simulink model "Modelo_NL_Ley_de_control_NL_EJE_Q"  (R2017a)
settings: Solver=VariableStepAuto  StartTime=0.0  StopTime=1  MaxStep=1e-4  RelTol=1e-3
values from neighbouring files (symbols this model uses):
  alfa_cu = 3.9e-3    (= 0.0039)    [modelo_global_NL.m]
  beq = bl/r^2 + bm    (= 1.5638971155e-05)    [Evaluacion_polos_5_2_2.m]    (also in modelo_global_NL.m = 1.5e-05)
  Cts = 0.818    [modelo_global_NL.m]
  Jeq = Jl/r^2 + Jm    (= 6.9338269301e-06)    [Evaluacion_polos_5_2_2.m]    (also in modelo_global_NL.m = 5.65588462007e-06)
  LambdaM = 0.01546    [Evaluacion_polos_5_2_2.m]    (also in modelo_global_NL.m)
  Ld = 0.0066    [Evaluacion_polos_5_2_2.m]    (also in modelo_global_NL.m)
  Lq = 0.0058    [Evaluacion_polos_5_2_2.m]    (also in modelo_global_NL.m)
  Pp = 3    [Evaluacion_polos_5_2_2.m]    (also in modelo_global_NL.m)
  Rsref = 1.02    [modelo_global_NL.m]
  Rts_amb = 146.7    [modelo_global_NL.m]
  Tamb = 40    [modelo_global_NL.m]
  Tleq = Tl/r    (= 0.02)    [modelo_global_NL.m]
  Tsref = 40    [modelo_global_NL.m]
  Vqs_nom = 19.596    [modelo_global_NL.m]
undefined symbols (not defined in the file or in its folder): sigbuilder_block
libraries: simulink x2
settings Model: Creator=merem  LastModifiedBy=merem

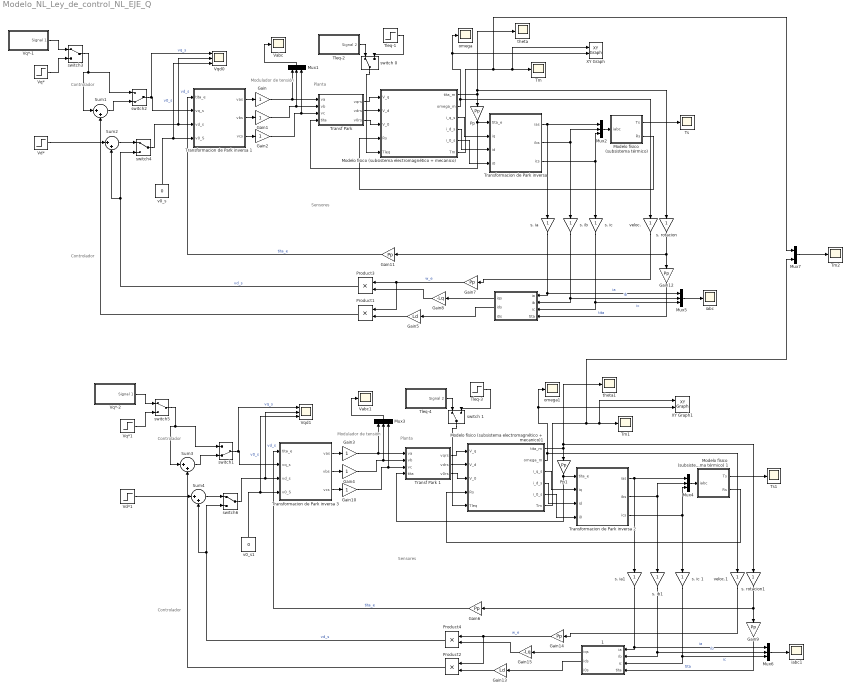
== system Modelo_NL_Ley_de_control_NL_EJE_Q ==
  note: Controlador
  note: Controlador
  note: Modulador de tensión
  note: Sensores
  note: Planta
  note: Controlador
  note: Modulador de tensión
  note: Controlador
  note: Sensores
  note: Planta
  " " : Subsystem
  " 1" : Subsystem
  Gain{,1..4,10} (6 alike) : Gain
  Gain{6..7,9,11..12,14} (6 alike) : Gain  Gain=Pp
  Gain13 : Gain  Gain=Ld
  Gain15 : Gain  Gain=-Lq
  Gain5 : Gain  Gain=Ld
  Gain8 : Gain  Gain=-Lq
  Modelo físico (subsistema electromagnético + mecanico) : Subsystem
  Modelo físico (subsistema electromagnético + mecanico)1 : Subsystem
  "Modelo físico (subsistema térmico) " : Subsystem
  Modelo físico (subsistema térmico) 1 : Subsystem
  Mux{1..6} (6 alike) : Mux  Inputs=3
  Mux7 : Mux  Inputs=2
  Pp : Gain  Gain=Pp
  Pp1 : Gain  Gain=Pp
  Product{1..4} (4 alike) : Product
  Sum{1..4} (4 alike) : Sum  Inputs=|++
  Tleq-1 : Step  Time=0.3  After=Tleq  SampleTime=0
  Tleq-2 : Subsystem  Tag=STV Subsys  LoadFcn=sigbuilder_block('load');  StartFcn=sigbuilder_block('start');  StopFcn=sigbuilder_block('stop');  ClipboardFcn=sigbuilder_block('clipboard');  mask(Sigbuilder block){tuvar=[0:10]}
      mask help: Simulink:masks:SigbuilderBlock_MD
      mask init:
      | if ~strcmp(get_param(bdroot(gcbh),'SimulationStatus'),'stopped') tuvar = sigbuilder_block('maskInit'); end
      settings: CopyFcn=sigbuilder_block('copy');  DeleteFcn=sigbuilder_block('delete');  ModelCloseFcn=sigbuilder_block('modelClose');  PreSaveFcn=sigbuilder_block('preSave');  PauseFcn=sigbuilder_block('pause');  ContinueFcn=sigbuilder_block('continue');  NameChangeFcn=sigbuilder_block('namechange');  OpenFcn=sigbuilder_block('open',[6 30 1012.5 447.75 ]);  CloseFcn=sigbuilder_block('close');
      mask Display: plot(0, 0, 100, 100,[2, 2, 32, 32, 2], [68, 8, 8, 68, 68],[32, 2], [38, 38], [32, 19, 2],[53, 60, 44], [32, 17, 17, 2],[16, 16, 31, 31]);txt = getActiveGroup(gcbh);text(2, 100, txt,'verticalAlignment', 'top');
  Tleq-3 : Step  Time=0.3  After=Tleq  SampleTime=0
  Tleq-4 : Subsystem  Tag=STV Subsys  LoadFcn=sigbuilder_block('load');  StartFcn=sigbuilder_block('start');  StopFcn=sigbuilder_block('stop');  ClipboardFcn=sigbuilder_block('clipboard');  mask(Sigbuilder block){tuvar=[0:10]}
      mask help: Simulink:masks:SigbuilderBlock_MD
      mask init:
      | if ~strcmp(get_param(bdroot(gcbh),'SimulationStatus'),'stopped') tuvar = sigbuilder_block('maskInit'); end
      settings: CopyFcn=sigbuilder_block('copy');  DeleteFcn=sigbuilder_block('delete');  ModelCloseFcn=sigbuilder_block('modelClose');  PreSaveFcn=sigbuilder_block('preSave');  PauseFcn=sigbuilder_block('pause');  ContinueFcn=sigbuilder_block('continue');  NameChangeFcn=sigbuilder_block('namechange');  OpenFcn=sigbuilder_block('open',[6 30 1012.5 447.75 ]);  CloseFcn=sigbuilder_block('close');
      mask Display: plot(0, 0, 100, 100,[2, 2, 32, 32, 2], [68, 8, 8, 68, 68],[32, 2], [38, 38], [32, 19, 2],[53, 60, 44], [32, 17, 17, 2],[16, 16, 31, 31]);txt = getActiveGroup(gcbh);text(2, 100, txt,'verticalAlignment', 'top');
  Tm : Scope
  Tm1 : Scope
  Tm2 : Scope
  "Transf Park " : Subsystem
  Transf Park 1 : Subsystem
  "Transformacion de Park inversa " : Subsystem
  Transformacion de Park inversa 1 : Subsystem
  Transformacion de Park inversa 2 : Subsystem
  Transformacion de Park inversa 3 : Subsystem
  Ts : Scope
  Ts1 : Scope
  Vabc : Scope
  Vabc1 : Scope
  Vd* : Step  Time=0.5  After=1.9596  SampleTime=0
  Vd*1 : Step  Time=0.5  After=1.9596  SampleTime=0
  Vq* : Step  Time=0.1  After=Vqs_nom  SampleTime=0
  Vq*-1 : Subsystem  Tag=STV Subsys  LoadFcn=sigbuilder_block('load');  StartFcn=sigbuilder_block('start');  StopFcn=sigbuilder_block('stop');  ClipboardFcn=sigbuilder_block('clipboard');  mask(Sigbuilder block){tuvar=[0:10]}
      mask help: Simulink:masks:SigbuilderBlock_MD
      mask init:
      | if ~strcmp(get_param(bdroot(gcbh),'SimulationStatus'),'stopped') tuvar = sigbuilder_block('maskInit'); end
      settings: CopyFcn=sigbuilder_block('copy');  DeleteFcn=sigbuilder_block('delete');  ModelCloseFcn=sigbuilder_block('modelClose');  PreSaveFcn=sigbuilder_block('preSave');  PauseFcn=sigbuilder_block('pause');  ContinueFcn=sigbuilder_block('continue');  NameChangeFcn=sigbuilder_block('namechange');  OpenFcn=sigbuilder_block('open',[6 -3.75 1012.5 407.25 ]);  CloseFcn=sigbuilder_block('close');
      mask Display: plot(0, 0, 100, 100,[2, 2, 32, 32, 2], [68, 8, 8, 68, 68],[32, 2], [38, 38], [32, 19, 2],[53, 60, 44], [32, 17, 17, 2],[16, 16, 31, 31]);txt = getActiveGroup(gcbh);text(2, 100, txt,'verticalAlignment', 'top');
  Vq*-2 : Subsystem  Tag=STV Subsys  LoadFcn=sigbuilder_block('load');  StartFcn=sigbuilder_block('start');  StopFcn=sigbuilder_block('stop');  ClipboardFcn=sigbuilder_block('clipboard');  mask(Sigbuilder block){tuvar=[0:10]}
      mask help: Simulink:masks:SigbuilderBlock_MD
      mask init:
      | if ~strcmp(get_param(bdroot(gcbh),'SimulationStatus'),'stopped') tuvar = sigbuilder_block('maskInit'); end
      settings: CopyFcn=sigbuilder_block('copy');  DeleteFcn=sigbuilder_block('delete');  ModelCloseFcn=sigbuilder_block('modelClose');  PreSaveFcn=sigbuilder_block('preSave');  PauseFcn=sigbuilder_block('pause');  ContinueFcn=sigbuilder_block('continue');  NameChangeFcn=sigbuilder_block('namechange');  OpenFcn=sigbuilder_block('open',[6 -3.75 1012.5 407.25 ]);  CloseFcn=sigbuilder_block('close');
      mask Display: plot(0, 0, 100, 100,[2, 2, 32, 32, 2], [68, 8, 8, 68, 68],[32, 2], [38, 38], [32, 19, 2],[53, 60, 44], [32, 17, 17, 2],[16, 16, 31, 31]);txt = getActiveGroup(gcbh);text(2, 100, txt,'verticalAlignment', 'top');
  Vq*1 : Step  Time=0.1  After=Vqs_nom  SampleTime=0
  Vqd0 : Scope  NumInputPorts=3
  Vqd1 : Scope  NumInputPorts=3
  XY Graph : simulink/Sinks/XY Graph  xmin=-0.6  xmax=0.6  ymin=-250  ymax=650  st=-1
  XY Graph1 : simulink/Sinks/XY Graph  xmin=-0.6  xmax=0.6  ymin=-250  ymax=650  st=-1
  iabc : Scope
  iabc1 : Scope
  omega : Scope
  omega1 : Scope
  s. ia : Gain
  s. ia1 : Gain
  s. ib : Gain
  s. ib1 : Gain
  "s. ic " : Gain
  s. ic 1 : Gain
  s. rotacion : Gain
  s. rotacion1 : Gain
  switch 0 : ManualSwitch
  switch 1 : ManualSwitch
  switch1 : ManualSwitch  CurrentSetting=0
  switch2 : ManualSwitch  CurrentSetting=0
  switch{3..6} (4 alike) : ManualSwitch
  theta : Scope
  theta1 : Scope
  v0_s : Constant  Value=0
  v0_s1 : Constant  Value=0
  veloc. : Gain
  veloc.1 : Gain
  wires:
  s. rotacion/1 -> Gain12/1, Gain11/1
  "s. ic "/1 -> Mux5/3, " "/3("ic ")  "ic"
  "Transformacion de Park inversa "/1(ias) -> s. ia/1, Mux2/1
  Gain/1 -> "Transf Park "/1("va "), Mux1/1
  Gain7/1 -> Product1/1, Product3/1  "w_e"
  Gain8/1 -> Product3/2
  Gain1/1 -> "Transf Park "/2(vb), Mux1/2
  s. ia/1 -> Mux5/1, " "/1("ia ")  "ia"
  Gain5/1 -> Product1/2
  Gain2/1 -> "Transf Park "/3(vc), Mux1/3
  Gain12/1 -> " "/4("tita ")  "tita"
  "Transformacion de Park inversa "/3("ics ") -> "s. ic "/1, Mux2/3
  v0_s/1 -> Vqd0/3, Transformacion de Park inversa 1/4("v0_S ")  "v0_s"
  Product3/1 -> Sum2/2, switch4/2  "vd_s"
  s. ib/1 -> Mux5/2, " "/2("ib ")  "ib"
  Gain11/1 -> Transformacion de Park inversa 1/1(tita_e)  "tita_e"
  " "/2("ids ") -> Gain5/1
  Transformacion de Park inversa 1/1(vas) -> Gain/1
  Transformacion de Park inversa 1/3("vcs ") -> Gain2/1
  " "/1(iqs) -> Gain8/1
  "Transformacion de Park inversa "/2(ibs) -> Mux2/2, s. ib/1
  Mux1/1 -> Vabc/1
  Transformacion de Park inversa 1/2(vbs) -> Gain1/1
  Product1/1 -> Sum1/2
  switch2/1 -> Vqd0/1, Transformacion de Park inversa 1/2(vq_s)  "vq_s"
  Sum1/1 -> switch2/2
  "Transf Park "/1(vqrs) -> Modelo físico (subsistema electromagnético + mecanico)/1(V_q)
  "Transf Park "/2("vdrs ") -> Modelo físico (subsistema electromagnético + mecanico)/2(V_d)
  "Transf Park "/3("v0rs ") -> Modelo físico (subsistema electromagnético + mecanico)/3(V_0)
  Pp/1 -> "Transf Park "/4(tita), "Transformacion de Park inversa "/1(tita_e)
  Modelo físico (subsistema electromagnético + mecanico)/1("tita_m ") -> s. rotacion/1, theta/1, Pp/1
  switch3/1 -> Sum1/1, switch2/1
  Vq*/1 -> switch3/2
  Vd*/1 -> Sum2/1
  switch4/1 -> Vqd0/2, Transformacion de Park inversa 1/3(vd_s)  "vd_s"
  Sum2/1 -> switch4/1
  Vq*-1/1(Signal 1) -> switch3/1
  Modelo físico (subsistema electromagnético + mecanico)/3("i_q_s ") -> "Transformacion de Park inversa "/2(iq)
  Modelo físico (subsistema electromagnético + mecanico)/4("i_d_s ") -> "Transformacion de Park inversa "/3(id)
  Modelo físico (subsistema electromagnético + mecanico)/5("i_0_s ") -> "Transformacion de Park inversa "/4(i0)
  Mux2/1 -> "Modelo físico (subsistema térmico) "/1(iabc)
  "Modelo físico (subsistema térmico) "/2(Rs) -> Modelo físico (subsistema electromagnético + mecanico)/4(Rs)
  Tleq-2/1(Signal 2) -> switch 0/1
  Tleq-1/1 -> switch 0/2
  switch 0/1 -> Modelo físico (subsistema electromagnético + mecanico)/5(Tleq)
  "Modelo físico (subsistema térmico) "/1(Ts) -> Ts/1
  Mux5/1 -> iabc/1
  Modelo físico (subsistema electromagnético + mecanico)/2("omega_m ") -> veloc./1, XY Graph/2, omega/1
  veloc./1 -> Gain7/1
  Modelo físico (subsistema electromagnético + mecanico)/6(Tm) -> Mux7/1, XY Graph/1, Tm/1
  Transformacion de Park inversa 2/2(ibs) -> Mux4/2, s. ib1/1
  Transformacion de Park inversa 2/1(ias) -> s. ia1/1, Mux4/1
  Transf Park 1/2("vdrs ") -> Modelo físico (subsistema electromagnético + mecanico)1/2(V_d)
  Transf Park 1/3("v0rs ") -> Modelo físico (subsistema electromagnético + mecanico)1/3(V_0)
  v0_s1/1 -> Vqd1/3, Transformacion de Park inversa 3/4("v0_S ")  "v0_s"
  Sum3/1 -> switch1/2
  Pp1/1 -> Transf Park 1/4(tita), Transformacion de Park inversa 2/1(tita_e)
  Transformacion de Park inversa 3/2(vbs) -> Gain4/1
  Gain14/1 -> Product2/1, Product4/1  "w_e"
  s. ib1/1 -> Mux6/2, " 1"/2("ib ")  "ib"
  Gain13/1 -> Product2/2
  Gain6/1 -> Transformacion de Park inversa 3/1(tita_e)  "tita_e"
  Gain3/1 -> Transf Park 1/1("va "), Mux3/1
  Gain4/1 -> Transf Park 1/2(vb), Mux3/2
  Tleq-3/1 -> switch 1/2
  Sum4/1 -> switch6/1
  Gain9/1 -> " 1"/4("tita ")  "tita"
  Product2/1 -> Sum3/2
  Transformacion de Park inversa 3/1(vas) -> Gain3/1
  Transformacion de Park inversa 3/3("vcs ") -> Gain10/1
  Modelo físico (subsistema electromagnético + mecanico)1/4("i_d_s ") -> Transformacion de Park inversa 2/3(id)
  " 1"/2("ids ") -> Gain13/1
  Mux3/1 -> Vabc1/1
  Tleq-4/1(Signal 2) -> switch 1/1
  switch6/1 -> Vqd1/2, Transformacion de Park inversa 3/3(vd_s)  "vd_s"
  Modelo físico (subsistema electromagnético + mecanico)1/1("tita_m ") -> s. rotacion1/1, theta1/1, Pp1/1
  switch5/1 -> Sum3/1, switch1/1
  Modelo físico (subsistema electromagnético + mecanico)1/3("i_q_s ") -> Transformacion de Park inversa 2/2(iq)
  Vq*-2/1(Signal 1) -> switch5/1
  Transf Park 1/1(vqrs) -> Modelo físico (subsistema electromagnético + mecanico)1/1(V_q)
  Gain15/1 -> Product4/2
  Modelo físico (subsistema térmico) 1/2(Rs) -> Modelo físico (subsistema electromagnético + mecanico)1/4(Rs)
  Product4/1 -> Sum4/2, switch6/2  "vd_s"
  switch 1/1 -> Modelo físico (subsistema electromagnético + mecanico)1/5(Tleq)
  s. ia1/1 -> Mux6/1, " 1"/1("ia ")  "ia"
  switch1/1 -> Vqd1/1, Transformacion de Park inversa 3/2(vq_s)  "vq_s"
  Modelo físico (subsistema térmico) 1/1(Ts) -> Ts1/1
  Modelo físico (subsistema electromagnético + mecanico)1/5("i_0_s ") -> Transformacion de Park inversa 2/4(i0)
  Transformacion de Park inversa 2/3("ics ") -> s. ic 1/1, Mux4/3
  Mux6/1 -> iabc1/1
  Vq*1/1 -> switch5/2
  " 1"/1(iqs) -> Gain15/1
  s. rotacion1/1 -> Gain9/1, Gain6/1
  Vd*1/1 -> Sum4/1
  Modelo físico (subsistema electromagnético + mecanico)1/2("omega_m ") -> veloc.1/1, XY Graph1/2, omega1/1
  s. ic 1/1 -> Mux6/3, " 1"/3("ic ")  "ic"
  Mux4/1 -> Modelo físico (subsistema térmico) 1/1(iabc)
  veloc.1/1 -> Gain14/1
  Gain10/1 -> Transf Park 1/3(vc), Mux3/3
  Mux7/1 -> Tm2/1
  Modelo físico (subsistema electromagnético + mecanico)1/6(Tm) -> Mux7/2, XY Graph1/1, Tm1/1

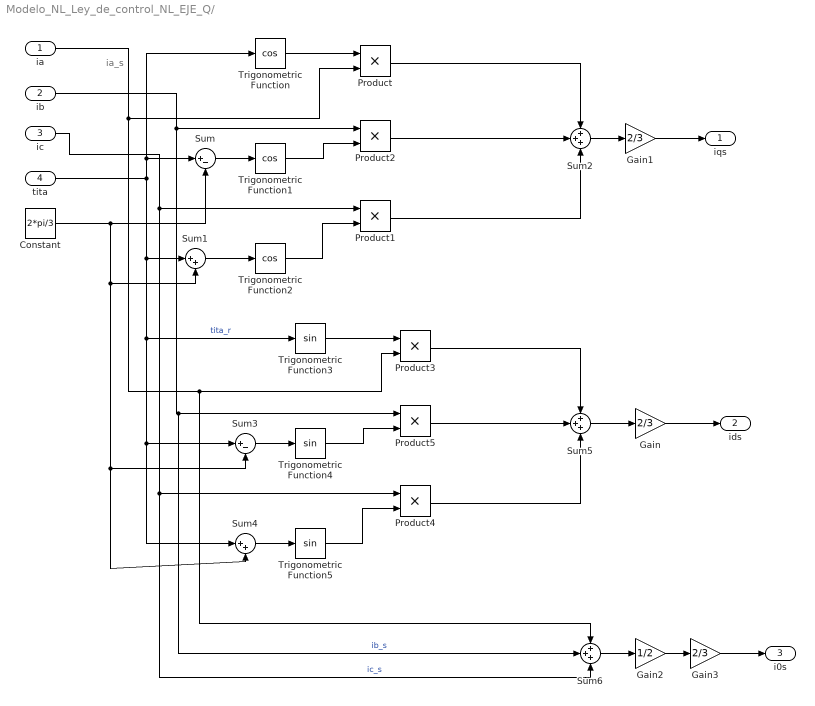
== system Modelo_NL_Ley_de_control_NL_EJE_Q/  ==
  note: ia_s
  "ia " : Inport
  "ib " : Inport  Port=2
  "ic " : Inport  Port=3
  "tita " : Inport  Port=4
  Constant : Constant  Value=2*pi/3
  Gain : Gain  Gain=2/3
  Gain1 : Gain  Gain=2/3
  Gain2 : Gain  Gain=1/2
  Gain3 : Gain  Gain=2/3
  Product{,1..5} (6 alike) : Product
  Sum : Sum  Inputs=|+-
  Sum1 : Sum  Inputs=|++
  Sum2 : Sum  Inputs=+++
  Sum3 : Sum  Inputs=|+-
  Sum4 : Sum  Inputs=|++
  Sum5 : Sum  Inputs=+++
  Sum6 : Sum  Inputs=+++
  Trigonometric Function : Trigonometry  Operator=cos
  Trigonometric Function1 : Trigonometry  Operator=cos
  Trigonometric Function2 : Trigonometry  Operator=cos
  Trigonometric Function3 : Trigonometry
  Trigonometric Function4 : Trigonometry
  Trigonometric Function5 : Trigonometry
  iqs : Outport
  "ids " : Outport  Port=2
  "i0s " : Outport  Port=3
  wires:
  "tita "/1 -> Trigonometric Function/1, Sum/1, Sum1/1, Trigonometric Function3/1, Sum3/1, Sum4/1  "tita_r"
  Trigonometric Function/1 -> Product/1
  "ia "/1 -> Sum6/1, Product3/2, Product/2
  Constant/1 -> Sum4/2, Sum3/2, Sum1/2, Sum/2
  Sum/1 -> Trigonometric Function1/1
  Sum1/1 -> Trigonometric Function2/1
  Trigonometric Function1/1 -> Product2/2
  Trigonometric Function2/1 -> Product1/2
  "ib "/1 -> Sum6/2, Product5/1, Product2/1  "ib_s"
  "ic "/1 -> Sum6/3, Product4/1, Product1/1  "ic_s"
  Product/1 -> Sum2/1
  Product2/1 -> Sum2/2
  Sum2/1 -> Gain1/1
  Trigonometric Function5/1 -> Product4/2
  Trigonometric Function3/1 -> Product3/1
  Sum4/1 -> Trigonometric Function5/1
  Sum3/1 -> Trigonometric Function4/1
  Trigonometric Function4/1 -> Product5/2
  Product3/1 -> Sum5/1
  Product5/1 -> Sum5/2
  Product4/1 -> Sum5/3
  Sum5/1 -> Gain/1
  Product1/1 -> Sum2/3
  Gain/1 -> "ids "/1
  Gain1/1 -> iqs/1
  Sum6/1 -> Gain2/1
  Gain2/1 -> Gain3/1
  Gain3/1 -> "i0s "/1

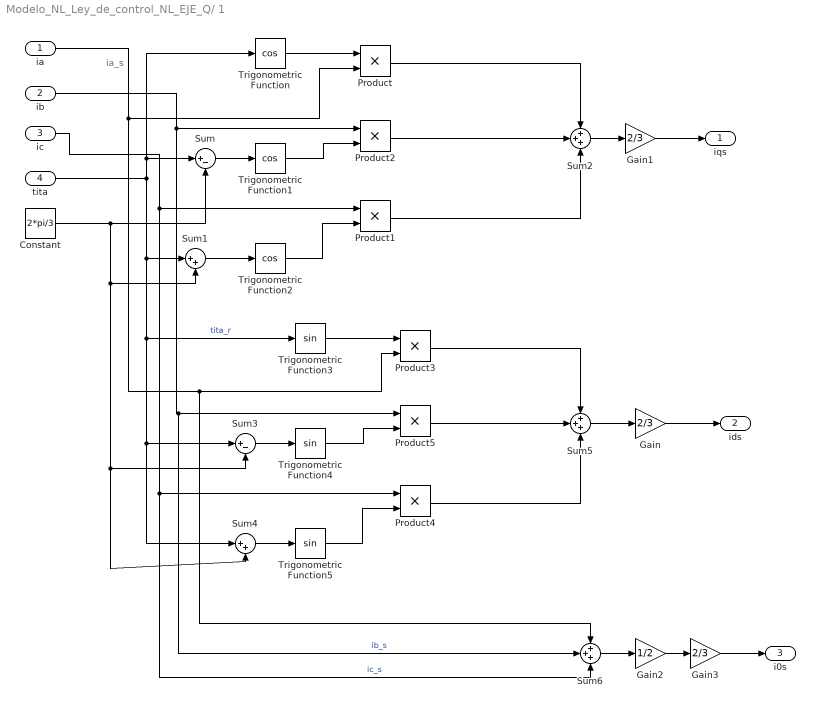
== system Modelo_NL_Ley_de_control_NL_EJE_Q/ 1 ==
  note: ia_s
  "ia " : Inport
  "ib " : Inport  Port=2
  "ic " : Inport  Port=3
  "tita " : Inport  Port=4
  Constant : Constant  Value=2*pi/3
  Gain : Gain  Gain=2/3
  Gain1 : Gain  Gain=2/3
  Gain2 : Gain  Gain=1/2
  Gain3 : Gain  Gain=2/3
  Product{,1..5} (6 alike) : Product
  Sum : Sum  Inputs=|+-
  Sum1 : Sum  Inputs=|++
  Sum2 : Sum  Inputs=+++
  Sum3 : Sum  Inputs=|+-
  Sum4 : Sum  Inputs=|++
  Sum5 : Sum  Inputs=+++
  Sum6 : Sum  Inputs=+++
  Trigonometric Function : Trigonometry  Operator=cos
  Trigonometric Function1 : Trigonometry  Operator=cos
  Trigonometric Function2 : Trigonometry  Operator=cos
  Trigonometric Function3 : Trigonometry
  Trigonometric Function4 : Trigonometry
  Trigonometric Function5 : Trigonometry
  iqs : Outport
  "ids " : Outport  Port=2
  "i0s " : Outport  Port=3
  wires:
  "tita "/1 -> Trigonometric Function/1, Sum/1, Sum1/1, Trigonometric Function3/1, Sum3/1, Sum4/1  "tita_r"
  Trigonometric Function/1 -> Product/1
  "ia "/1 -> Sum6/1, Product3/2, Product/2
  Constant/1 -> Sum4/2, Sum3/2, Sum1/2, Sum/2
  Sum/1 -> Trigonometric Function1/1
  Sum1/1 -> Trigonometric Function2/1
  Trigonometric Function1/1 -> Product2/2
  Trigonometric Function2/1 -> Product1/2
  "ib "/1 -> Sum6/2, Product5/1, Product2/1  "ib_s"
  "ic "/1 -> Sum6/3, Product4/1, Product1/1  "ic_s"
  Product/1 -> Sum2/1
  Product2/1 -> Sum2/2
  Sum2/1 -> Gain1/1
  Trigonometric Function5/1 -> Product4/2
  Trigonometric Function3/1 -> Product3/1
  Sum4/1 -> Trigonometric Function5/1
  Sum3/1 -> Trigonometric Function4/1
  Trigonometric Function4/1 -> Product5/2
  Product3/1 -> Sum5/1
  Product5/1 -> Sum5/2
  Product4/1 -> Sum5/3
  Sum5/1 -> Gain/1
  Product1/1 -> Sum2/3
  Gain/1 -> "ids "/1
  Gain1/1 -> iqs/1
  Sum6/1 -> Gain2/1
  Gain2/1 -> Gain3/1
  Gain3/1 -> "i0s "/1

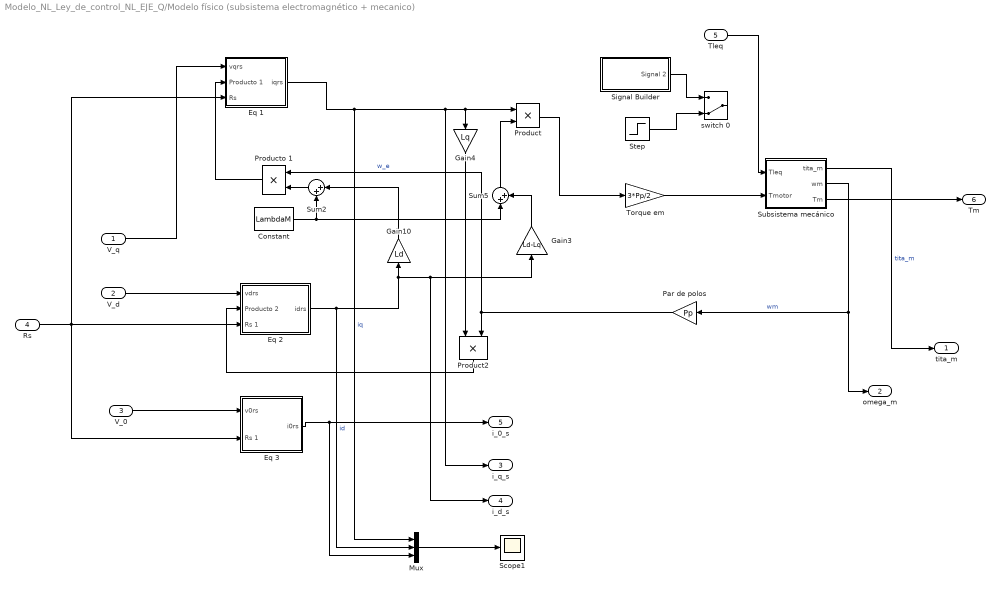
== system Modelo_NL_Ley_de_control_NL_EJE_Q/Modelo físico (subsistema electromagnético + mecanico) ==
  V_q : Inport
  V_d : Inport  Port=2
  V_0 : Inport  Port=3
  Rs : Inport  Port=4
  Tleq : Inport  Port=5
  Constant : Constant  Value=LambdaM
  Eq 1 : Subsystem
  "Eq 2 " : Subsystem
  Eq 3 : Subsystem
  Gain10 : Gain  Gain=Ld
  Gain3 : Gain  Gain=Ld-Lq
  Gain4 : Gain  Gain=Lq
  Mux : Mux  Inputs=3
  Par de polos : Gain  Gain=Pp
  Product : Product
  Product2 : Product
  Producto 1 : Product
  Scope1 : Scope
  Signal Builder : Subsystem  Tag=STV Subsys  LoadFcn=sigbuilder_block('load');  StartFcn=sigbuilder_block('start');  StopFcn=sigbuilder_block('stop');  ClipboardFcn=sigbuilder_block('clipboard');  mask(Sigbuilder block){tuvar=[0:10]}
      mask help: Simulink:masks:SigbuilderBlock_MD
      mask init:
      | if ~strcmp(get_param(bdroot(gcbh),'SimulationStatus'),'stopped') tuvar = sigbuilder_block('maskInit'); end
      settings: CopyFcn=sigbuilder_block('copy');  DeleteFcn=sigbuilder_block('delete');  ModelCloseFcn=sigbuilder_block('modelClose');  PreSaveFcn=sigbuilder_block('preSave');  PauseFcn=sigbuilder_block('pause');  ContinueFcn=sigbuilder_block('continue');  NameChangeFcn=sigbuilder_block('namechange');  OpenFcn=sigbuilder_block('open',[6 30 1012.5 447.75 ]);  CloseFcn=sigbuilder_block('close');
      mask Display: plot(0, 0, 100, 100,[2, 2, 32, 32, 2], [68, 8, 8, 68, 68],[32, 2], [38, 38], [32, 19, 2],[53, 60, 44], [32, 17, 17, 2],[16, 16, 31, 31]);txt = getActiveGroup(gcbh);text(2, 100, txt,'verticalAlignment', 'top');
  Step : Step  Time=0.3  After=Tleq  SampleTime=0
  Subsistema mecánico : Subsystem
  Sum2 : Sum  Inputs=|++
  Sum5 : Sum  Inputs=|++
  "Torque em " : Gain  Gain=3*Pp/2
  switch 0 : ManualSwitch  CurrentSetting=0
  "tita_m " : Outport
  "omega_m " : Outport  Port=2
  "i_q_s " : Outport  Port=3
  "i_d_s " : Outport  Port=4
  "i_0_s " : Outport  Port=5
  Tm : Outport  Port=6
  wires:
  Sum2/1 -> Producto 1/2
  Sum5/1 -> Product/2
  Subsistema mecánico/2("wm ") -> "omega_m "/1, Par de polos/1  "wm"
  V_q/1 -> Eq 1/1(vqrs)
  Gain10/1 -> Sum2/1
  Par de polos/1 -> Producto 1/1, Product2/2  "w_e"
  "Torque em "/1 -> Subsistema mecánico/2("Tmotor ")
  Product/1 -> "Torque em "/1
  Constant/1 -> Sum5/1, Sum2/2
  Gain3/1 -> Sum5/2
  Gain4/1 -> Product2/1
  Eq 1/1("iqrs ") -> Mux/1, "i_q_s "/1, Gain4/1, Product/1  "iq"
  Subsistema mecánico/1("tita_m ") -> "tita_m "/1  "tita_m"
  "Eq 2 "/1("idrs ") -> Mux/2, "i_d_s "/1, Gain3/1, Gain10/1  "id"
  Product2/1 -> "Eq 2 "/2("Producto 2 ")
  Producto 1/1 -> Eq 1/2("Producto 1 ")
  V_d/1 -> "Eq 2 "/1("vdrs ")
  V_0/1 -> Eq 3/1("v0rs ")
  Eq 3/1("i0rs ") -> Mux/3, "i_0_s "/1
  Step/1 -> switch 0/2
  Signal Builder/1(Signal 2) -> switch 0/1
  Rs/1 -> "Eq 2 "/3(Rs 1), Eq 3/2(Rs 1), Eq 1/3(Rs)
  Mux/1 -> Scope1/1
  Subsistema mecánico/3(Tm) -> Tm/1
  Tleq/1 -> Subsistema mecánico/1("Tleq ")

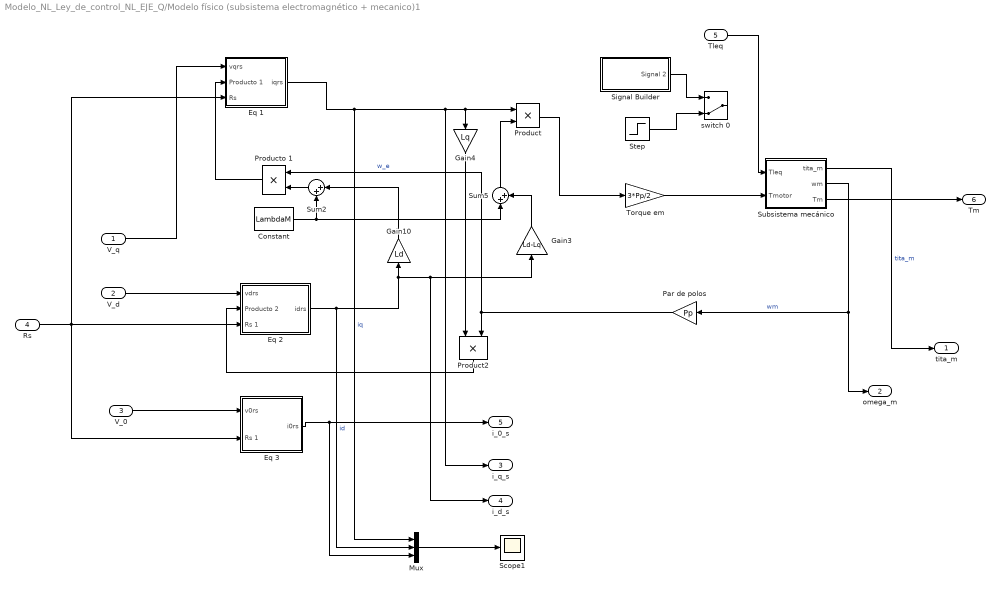
== system Modelo_NL_Ley_de_control_NL_EJE_Q/Modelo físico (subsistema electromagnético + mecanico)1 ==
  V_q : Inport
  V_d : Inport  Port=2
  V_0 : Inport  Port=3
  Rs : Inport  Port=4
  Tleq : Inport  Port=5
  Constant : Constant  Value=LambdaM
  Eq 1 : Subsystem
  "Eq 2 " : Subsystem
  Eq 3 : Subsystem
  Gain10 : Gain  Gain=Ld
  Gain3 : Gain  Gain=Ld-Lq
  Gain4 : Gain  Gain=Lq
  Mux : Mux  Inputs=3
  Par de polos : Gain  Gain=Pp
  Product : Product
  Product2 : Product
  Producto 1 : Product
  Scope1 : Scope
  Signal Builder : Subsystem  Tag=STV Subsys  LoadFcn=sigbuilder_block('load');  StartFcn=sigbuilder_block('start');  StopFcn=sigbuilder_block('stop');  ClipboardFcn=sigbuilder_block('clipboard');  mask(Sigbuilder block){tuvar=[0:10]}
      mask help: Simulink:masks:SigbuilderBlock_MD
      mask init:
      | if ~strcmp(get_param(bdroot(gcbh),'SimulationStatus'),'stopped') tuvar = sigbuilder_block('maskInit'); end
      settings: CopyFcn=sigbuilder_block('copy');  DeleteFcn=sigbuilder_block('delete');  ModelCloseFcn=sigbuilder_block('modelClose');  PreSaveFcn=sigbuilder_block('preSave');  PauseFcn=sigbuilder_block('pause');  ContinueFcn=sigbuilder_block('continue');  NameChangeFcn=sigbuilder_block('namechange');  OpenFcn=sigbuilder_block('open',[6 30 1012.5 447.75 ]);  CloseFcn=sigbuilder_block('close');
      mask Display: plot(0, 0, 100, 100,[2, 2, 32, 32, 2], [68, 8, 8, 68, 68],[32, 2], [38, 38], [32, 19, 2],[53, 60, 44], [32, 17, 17, 2],[16, 16, 31, 31]);txt = getActiveGroup(gcbh);text(2, 100, txt,'verticalAlignment', 'top');
  Step : Step  Time=0.3  After=Tleq  SampleTime=0
  Subsistema mecánico : Subsystem
  Sum2 : Sum  Inputs=|++
  Sum5 : Sum  Inputs=|++
  "Torque em " : Gain  Gain=3*Pp/2
  switch 0 : ManualSwitch  CurrentSetting=0
  "tita_m " : Outport
  "omega_m " : Outport  Port=2
  "i_q_s " : Outport  Port=3
  "i_d_s " : Outport  Port=4
  "i_0_s " : Outport  Port=5
  Tm : Outport  Port=6
  wires:
  Sum2/1 -> Producto 1/2
  Sum5/1 -> Product/2
  Subsistema mecánico/2("wm ") -> "omega_m "/1, Par de polos/1  "wm"
  V_q/1 -> Eq 1/1(vqrs)
  Gain10/1 -> Sum2/1
  Par de polos/1 -> Producto 1/1, Product2/2  "w_e"
  "Torque em "/1 -> Subsistema mecánico/2("Tmotor ")
  Product/1 -> "Torque em "/1
  Constant/1 -> Sum5/1, Sum2/2
  Gain3/1 -> Sum5/2
  Gain4/1 -> Product2/1
  Eq 1/1("iqrs ") -> Mux/1, "i_q_s "/1, Gain4/1, Product/1  "iq"
  Subsistema mecánico/1("tita_m ") -> "tita_m "/1  "tita_m"
  "Eq 2 "/1("idrs ") -> Mux/2, "i_d_s "/1, Gain3/1, Gain10/1  "id"
  Product2/1 -> "Eq 2 "/2("Producto 2 ")
  Producto 1/1 -> Eq 1/2("Producto 1 ")
  V_d/1 -> "Eq 2 "/1("vdrs ")
  V_0/1 -> Eq 3/1("v0rs ")
  Eq 3/1("i0rs ") -> Mux/3, "i_0_s "/1
  Step/1 -> switch 0/2
  Signal Builder/1(Signal 2) -> switch 0/1
  Rs/1 -> "Eq 2 "/3(Rs 1), Eq 3/2(Rs 1), Eq 1/3(Rs)
  Mux/1 -> Scope1/1
  Subsistema mecánico/3(Tm) -> Tm/1
  Tleq/1 -> Subsistema mecánico/1("Tleq ")

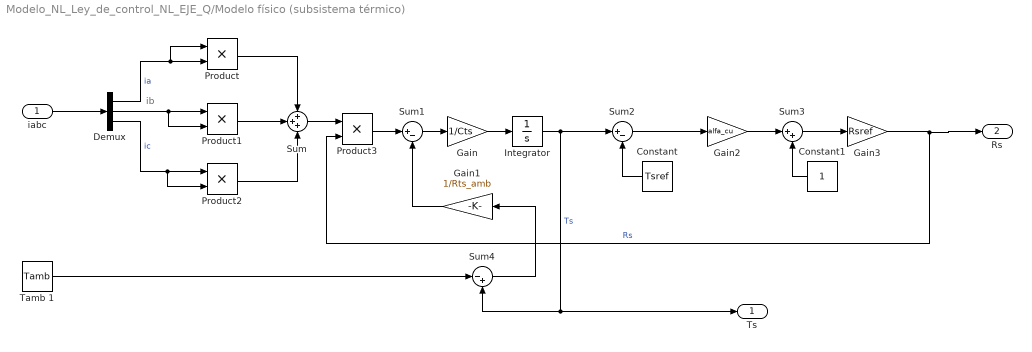
== system Modelo_NL_Ley_de_control_NL_EJE_Q/Modelo físico (subsistema térmico)  ==
  note: ib
  iabc : Inport
  Constant : Constant  Value=Tsref
  Constant1 : Constant
  Demux : Demux  Outputs=3
  Gain : Gain  Gain=1/Cts
  Gain1 : Gain  Gain=1/Rts_amb
  Gain2 : Gain  Gain=alfa_cu
  Gain3 : Gain  Gain=Rsref
  Integrator : Integrator  InitialCondition=40
  Product{,1..3} (4 alike) : Product
  Sum : Sum  Inputs=+++
  Sum1 : Sum  Inputs=|+-
  Sum2 : Sum  Inputs=|+-
  Sum3 : Sum  Inputs=|++
  Sum4 : Sum  Inputs=|-+
  Tamb 1 : Constant  Value=Tamb
  Ts : Outport
  Rs : Outport  Port=2
  wires:
  iabc/1 -> Demux/1
  Demux/1 -> Product/2, Product/1  "ia"
  Demux/2 -> Product1/2, Product1/1
  Demux/3 -> Product2/2, Product2/1  "ic"
  Product/1 -> Sum/1
  Product1/1 -> Sum/2
  Product2/1 -> Sum/3
  Sum/1 -> Product3/1
  Gain/1 -> Integrator/1
  Product3/1 -> Sum1/1
  Sum1/1 -> Gain/1
  Gain1/1 -> Sum1/2
  Integrator/1 -> Ts/1, Sum4/2, Sum2/1  "Ts"
  Constant/1 -> Sum2/2
  Sum2/1 -> Gain2/1
  Gain2/1 -> Sum3/1
  Constant1/1 -> Sum3/2
  Sum3/1 -> Gain3/1
  Gain3/1 -> Rs/1, Product3/2  "Rs"
  Tamb 1/1 -> Sum4/1
  Sum4/1 -> Gain1/1

== system Modelo_NL_Ley_de_control_NL_EJE_Q/Modelo físico (subsistema térmico) 1 ==
  note: ib
  iabc : Inport
  Constant : Constant  Value=Tsref
  Constant1 : Constant
  Demux : Demux  Outputs=3
  Gain : Gain  Gain=1/Cts
  Gain1 : Gain  Gain=1/Rts_amb
  Gain2 : Gain  Gain=alfa_cu
  Gain3 : Gain  Gain=Rsref
  Integrator : Integrator  InitialCondition=40
  Product{,1..3} (4 alike) : Product
  Sum : Sum  Inputs=+++
  Sum1 : Sum  Inputs=|+-
  Sum2 : Sum  Inputs=|+-
  Sum3 : Sum  Inputs=|++
  Sum4 : Sum  Inputs=|-+
  Tamb 1 : Constant  Value=Tamb
  Ts : Outport
  Rs : Outport  Port=2
  wires:
  iabc/1 -> Demux/1
  Demux/1 -> Product/2, Product/1  "ia"
  Demux/2 -> Product1/2, Product1/1
  Demux/3 -> Product2/2, Product2/1  "ic"
  Product/1 -> Sum/1
  Product1/1 -> Sum/2
  Product2/1 -> Sum/3
  Sum/1 -> Product3/1
  Gain/1 -> Integrator/1
  Product3/1 -> Sum1/1
  Sum1/1 -> Gain/1
  Gain1/1 -> Sum1/2
  Integrator/1 -> Ts/1, Sum4/2, Sum2/1  "Ts"
  Constant/1 -> Sum2/2
  Sum2/1 -> Gain2/1
  Gain2/1 -> Sum3/1
  Constant1/1 -> Sum3/2
  Sum3/1 -> Gain3/1
  Gain3/1 -> Rs/1, Product3/2  "Rs"
  Tamb 1/1 -> Sum4/1
  Sum4/1 -> Gain1/1

== system Modelo_NL_Ley_de_control_NL_EJE_Q/Tleq-2 ==
  Demux : Demux  Tag=STV Demux  Outputs=1
  FromWs : FromWorkspace  Tag=STV FromWs  VariableName=tuvar  SampleTime=0
      SigBuilderData=|
      | common.afterFinalStr = 'Extrapolate'
      | common.sampleTime = 0
      | dataSet.timeRange = [0 2]
      | dataSet.name = 'Group 1'
      | sbobj.Groups.Name = 'Group 1'
      | sbobj.Groups.Signals.Name = 'Signal 2'
      | sbobj.Groups.Signals.XData = [0 0.3 0.3 0.5 0.5 0.9 0.9 2]
      | sbobj.Groups.Signals.YData = [0 0 0.02 0.02 -0.02 -0.02 0 0]
      | sbobj.Groups.TimeRange = [0 2]
  Signal 2 : Outport  Tag=STV Outport
  wires:
  FromWs/1 -> Demux/1
  Demux/1 -> Signal 2/1

== system Modelo_NL_Ley_de_control_NL_EJE_Q/Tleq-4 ==
  Demux : Demux  Tag=STV Demux  Outputs=1
  FromWs : FromWorkspace  Tag=STV FromWs  VariableName=tuvar  SampleTime=0
      SigBuilderData=|
      | common.afterFinalStr = 'Extrapolate'
      | common.sampleTime = 0
      | dataSet.timeRange = [0 2]
      | dataSet.name = 'Group 1'
      | sbobj.Groups.Name = 'Group 1'
      | sbobj.Groups.Signals.Name = 'Signal 2'
      | sbobj.Groups.Signals.XData = [0 0.3 0.3 0.5 0.5 0.9 0.9 2]
      | sbobj.Groups.Signals.YData = [0 0 0.02 0.02 -0.02 -0.02 0 0]
      | sbobj.Groups.TimeRange = [0 2]
  Signal 2 : Outport  Tag=STV Outport
  wires:
  FromWs/1 -> Demux/1
  Demux/1 -> Signal 2/1

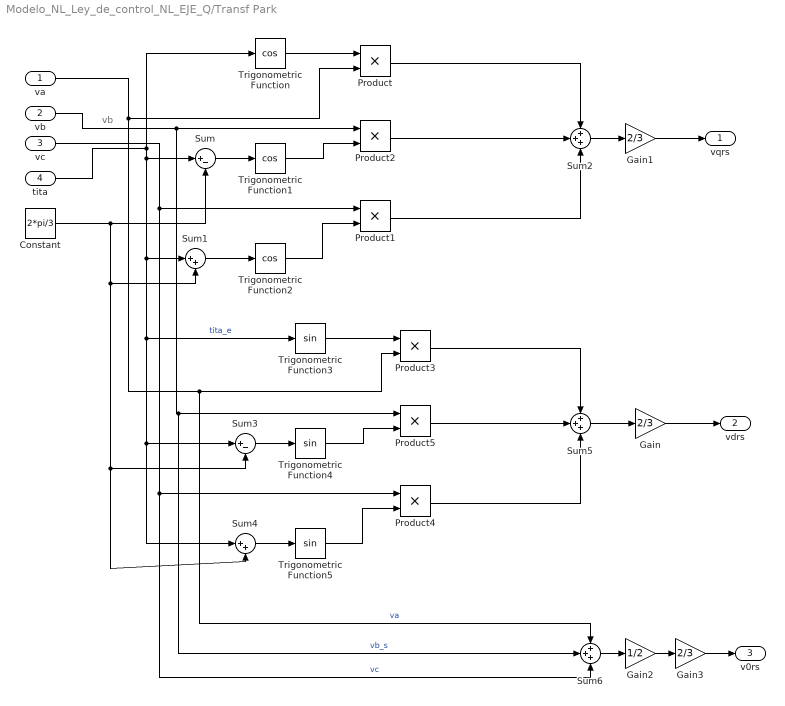
== system Modelo_NL_Ley_de_control_NL_EJE_Q/Transf Park  ==
  note: vb
  "va " : Inport
  vb : Inport  Port=2
  vc : Inport  Port=3
  tita : Inport  Port=4
  Constant : Constant  Value=2*pi/3
  Gain : Gain  Gain=2/3
  Gain1 : Gain  Gain=2/3
  Gain2 : Gain  Gain=1/2
  Gain3 : Gain  Gain=2/3
  Product{,1..5} (6 alike) : Product
  Sum : Sum  Inputs=|+-
  Sum1 : Sum  Inputs=|++
  Sum2 : Sum  Inputs=+++
  Sum3 : Sum  Inputs=|+-
  Sum4 : Sum  Inputs=|++
  Sum5 : Sum  Inputs=+++
  Sum6 : Sum  Inputs=+++
  Trigonometric Function : Trigonometry  Operator=cos
  Trigonometric Function1 : Trigonometry  Operator=cos
  Trigonometric Function2 : Trigonometry  Operator=cos
  Trigonometric Function3 : Trigonometry
  Trigonometric Function4 : Trigonometry
  Trigonometric Function5 : Trigonometry
  vqrs : Outport
  "vdrs " : Outport  Port=2
  "v0rs " : Outport  Port=3
  wires:
  tita/1 -> Sum1/1, Trigonometric Function3/1, Sum3/1, Sum4/1, Sum/1, Trigonometric Function/1  "tita_e"
  Trigonometric Function/1 -> Product/1
  "va "/1 -> Sum6/1, Product3/2, Product/2  "va"
  Constant/1 -> Sum4/2, Sum3/2, Sum1/2, Sum/2
  Sum/1 -> Trigonometric Function1/1
  Sum1/1 -> Trigonometric Function2/1
  Trigonometric Function1/1 -> Product2/2
  Trigonometric Function2/1 -> Product1/2
  vb/1 -> Sum6/2, Product5/1, Product2/1  "vb_s"
  vc/1 -> Sum6/3, Product4/1, Product1/1  "vc"
  Product/1 -> Sum2/1
  Product2/1 -> Sum2/2
  Sum2/1 -> Gain1/1
  Trigonometric Function5/1 -> Product4/2
  Trigonometric Function3/1 -> Product3/1
  Sum4/1 -> Trigonometric Function5/1
  Sum3/1 -> Trigonometric Function4/1
  Trigonometric Function4/1 -> Product5/2
  Product3/1 -> Sum5/1
  Product5/1 -> Sum5/2
  Product4/1 -> Sum5/3
  Sum5/1 -> Gain/1
  Product1/1 -> Sum2/3
  Gain/1 -> "vdrs "/1
  Gain1/1 -> vqrs/1
  Sum6/1 -> Gain2/1
  Gain3/1 -> "v0rs "/1
  Gain2/1 -> Gain3/1

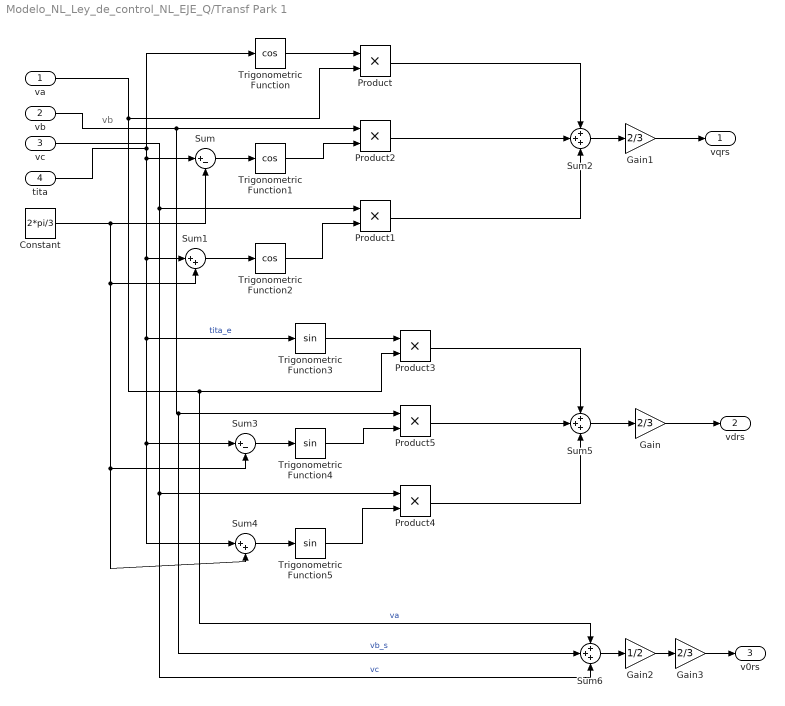
== system Modelo_NL_Ley_de_control_NL_EJE_Q/Transf Park 1 ==
  note: vb
  "va " : Inport
  vb : Inport  Port=2
  vc : Inport  Port=3
  tita : Inport  Port=4
  Constant : Constant  Value=2*pi/3
  Gain : Gain  Gain=2/3
  Gain1 : Gain  Gain=2/3
  Gain2 : Gain  Gain=1/2
  Gain3 : Gain  Gain=2/3
  Product{,1..5} (6 alike) : Product
  Sum : Sum  Inputs=|+-
  Sum1 : Sum  Inputs=|++
  Sum2 : Sum  Inputs=+++
  Sum3 : Sum  Inputs=|+-
  Sum4 : Sum  Inputs=|++
  Sum5 : Sum  Inputs=+++
  Sum6 : Sum  Inputs=+++
  Trigonometric Function : Trigonometry  Operator=cos
  Trigonometric Function1 : Trigonometry  Operator=cos
  Trigonometric Function2 : Trigonometry  Operator=cos
  Trigonometric Function3 : Trigonometry
  Trigonometric Function4 : Trigonometry
  Trigonometric Function5 : Trigonometry
  vqrs : Outport
  "vdrs " : Outport  Port=2
  "v0rs " : Outport  Port=3
  wires:
  tita/1 -> Sum1/1, Trigonometric Function3/1, Sum3/1, Sum4/1, Sum/1, Trigonometric Function/1  "tita_e"
  Trigonometric Function/1 -> Product/1
  "va "/1 -> Sum6/1, Product3/2, Product/2  "va"
  Constant/1 -> Sum4/2, Sum3/2, Sum1/2, Sum/2
  Sum/1 -> Trigonometric Function1/1
  Sum1/1 -> Trigonometric Function2/1
  Trigonometric Function1/1 -> Product2/2
  Trigonometric Function2/1 -> Product1/2
  vb/1 -> Sum6/2, Product5/1, Product2/1  "vb_s"
  vc/1 -> Sum6/3, Product4/1, Product1/1  "vc"
  Product/1 -> Sum2/1
  Product2/1 -> Sum2/2
  Sum2/1 -> Gain1/1
  Trigonometric Function5/1 -> Product4/2
  Trigonometric Function3/1 -> Product3/1
  Sum4/1 -> Trigonometric Function5/1
  Sum3/1 -> Trigonometric Function4/1
  Trigonometric Function4/1 -> Product5/2
  Product3/1 -> Sum5/1
  Product5/1 -> Sum5/2
  Product4/1 -> Sum5/3
  Sum5/1 -> Gain/1
  Product1/1 -> Sum2/3
  Gain/1 -> "vdrs "/1
  Gain1/1 -> vqrs/1
  Sum6/1 -> Gain2/1
  Gain3/1 -> "v0rs "/1
  Gain2/1 -> Gain3/1

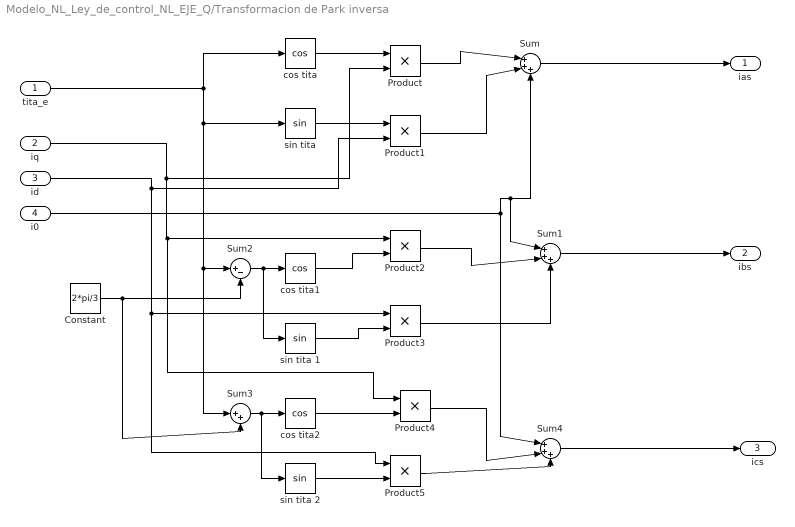
== system Modelo_NL_Ley_de_control_NL_EJE_Q/Transformacion de Park inversa  ==
  tita_e : Inport
  iq : Inport  Port=2
  id : Inport  Port=3
  i0 : Inport  Port=4
  Constant : Constant  Value=2*pi/3
  Product{,1..5} (6 alike) : Product
  Sum : Sum  Inputs=|+++
  Sum1 : Sum  Inputs=|+++
  Sum2 : Sum  Inputs=|+-
  Sum3 : Sum  Inputs=|++
  Sum4 : Sum  Inputs=|+++
  cos tita : Trigonometry  Operator=cos
  cos tita1 : Trigonometry  Operator=cos
  cos tita2 : Trigonometry  Operator=cos
  "sin tita " : Trigonometry
  sin tita 1 : Trigonometry
  sin tita 2 : Trigonometry
  ias : Outport
  ibs : Outport  Port=2
  "ics " : Outport  Port=3
  wires:
  tita_e/1 -> Sum3/1, Sum2/1, "sin tita "/1, cos tita/1
  iq/1 -> Product4/1, Product2/1, Product/2
  cos tita/1 -> Product/1
  "sin tita "/1 -> Product1/1
  id/1 -> Product5/1, Product3/1, Product1/2
  Product/1 -> Sum/1
  Product1/1 -> Sum/2
  Sum/1 -> ias/1
  i0/1 -> Sum1/1, Sum/3, Sum4/1
  cos tita1/1 -> Product2/2
  sin tita 1/1 -> Product3/2
  Product3/1 -> Sum1/3
  Product2/1 -> Sum1/2
  Sum1/1 -> ibs/1
  Constant/1 -> Sum3/2, Sum2/2
  Sum2/1 -> sin tita 1/1, cos tita1/1
  Sum3/1 -> sin tita 2/1, cos tita2/1
  cos tita2/1 -> Product4/2
  sin tita 2/1 -> Product5/2
  Product5/1 -> Sum4/3
  Product4/1 -> Sum4/2
  Sum4/1 -> "ics "/1

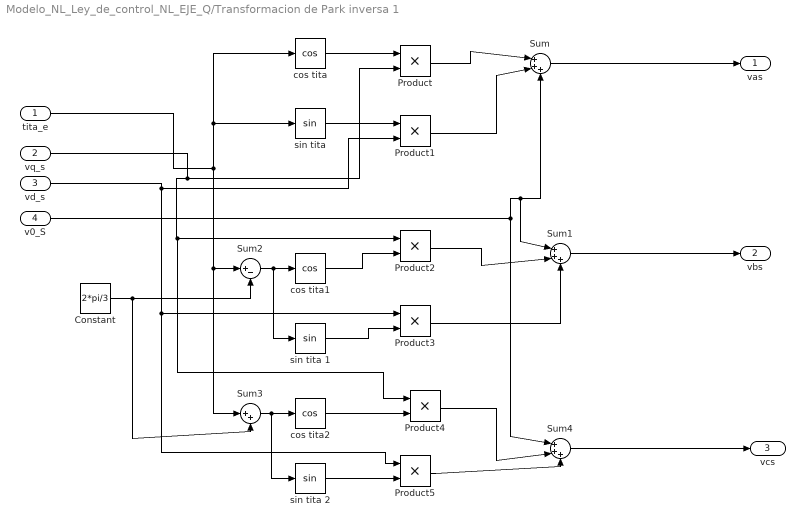
== system Modelo_NL_Ley_de_control_NL_EJE_Q/Transformacion de Park inversa 1 ==
  tita_e : Inport
  vq_s : Inport  Port=2
  vd_s : Inport  Port=3
  "v0_S " : Inport  Port=4
  Constant : Constant  Value=2*pi/3
  Product{,1..5} (6 alike) : Product
  Sum : Sum  Inputs=|+++
  Sum1 : Sum  Inputs=|+++
  Sum2 : Sum  Inputs=|+-
  Sum3 : Sum  Inputs=|++
  Sum4 : Sum  Inputs=|+++
  cos tita : Trigonometry  Operator=cos
  cos tita1 : Trigonometry  Operator=cos
  cos tita2 : Trigonometry  Operator=cos
  "sin tita " : Trigonometry
  sin tita 1 : Trigonometry
  sin tita 2 : Trigonometry
  vas : Outport
  vbs : Outport  Port=2
  "vcs " : Outport  Port=3
  wires:
  tita_e/1 -> Sum3/1, Sum2/1, cos tita/1, "sin tita "/1
  vq_s/1 -> Product4/1, Product2/1, Product/2
  cos tita/1 -> Product/1
  "sin tita "/1 -> Product1/1
  vd_s/1 -> Product5/1, Product3/1, Product1/2
  Product/1 -> Sum/1
  Product1/1 -> Sum/2
  Sum/1 -> vas/1
  "v0_S "/1 -> Sum1/1, Sum/3, Sum4/1
  cos tita1/1 -> Product2/2
  sin tita 1/1 -> Product3/2
  Product3/1 -> Sum1/3
  Product2/1 -> Sum1/2
  Sum1/1 -> vbs/1
  Constant/1 -> Sum3/2, Sum2/2
  Sum2/1 -> sin tita 1/1, cos tita1/1
  Sum3/1 -> sin tita 2/1, cos tita2/1
  cos tita2/1 -> Product4/2
  sin tita 2/1 -> Product5/2
  Product5/1 -> Sum4/3
  Product4/1 -> Sum4/2
  Sum4/1 -> "vcs "/1

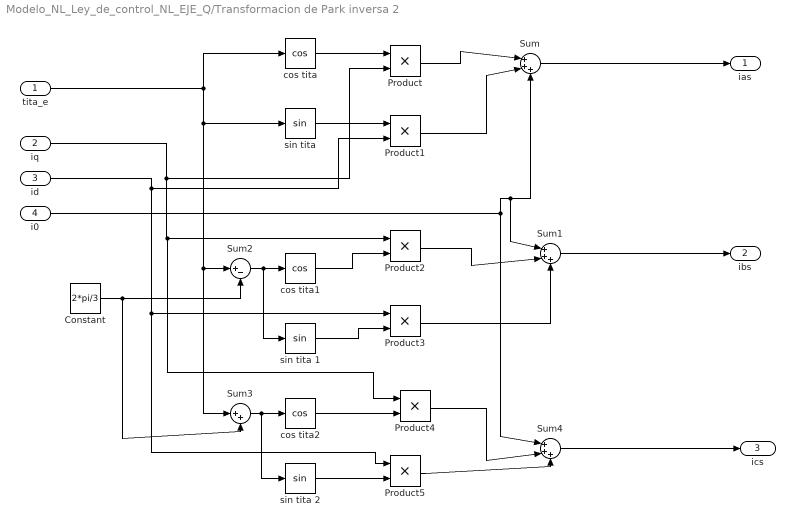
== system Modelo_NL_Ley_de_control_NL_EJE_Q/Transformacion de Park inversa 2 ==
  tita_e : Inport
  iq : Inport  Port=2
  id : Inport  Port=3
  i0 : Inport  Port=4
  Constant : Constant  Value=2*pi/3
  Product{,1..5} (6 alike) : Product
  Sum : Sum  Inputs=|+++
  Sum1 : Sum  Inputs=|+++
  Sum2 : Sum  Inputs=|+-
  Sum3 : Sum  Inputs=|++
  Sum4 : Sum  Inputs=|+++
  cos tita : Trigonometry  Operator=cos
  cos tita1 : Trigonometry  Operator=cos
  cos tita2 : Trigonometry  Operator=cos
  "sin tita " : Trigonometry
  sin tita 1 : Trigonometry
  sin tita 2 : Trigonometry
  ias : Outport
  ibs : Outport  Port=2
  "ics " : Outport  Port=3
  wires:
  tita_e/1 -> Sum3/1, Sum2/1, "sin tita "/1, cos tita/1
  iq/1 -> Product4/1, Product2/1, Product/2
  cos tita/1 -> Product/1
  "sin tita "/1 -> Product1/1
  id/1 -> Product5/1, Product3/1, Product1/2
  Product/1 -> Sum/1
  Product1/1 -> Sum/2
  Sum/1 -> ias/1
  i0/1 -> Sum1/1, Sum/3, Sum4/1
  cos tita1/1 -> Product2/2
  sin tita 1/1 -> Product3/2
  Product3/1 -> Sum1/3
  Product2/1 -> Sum1/2
  Sum1/1 -> ibs/1
  Constant/1 -> Sum3/2, Sum2/2
  Sum2/1 -> sin tita 1/1, cos tita1/1
  Sum3/1 -> sin tita 2/1, cos tita2/1
  cos tita2/1 -> Product4/2
  sin tita 2/1 -> Product5/2
  Product5/1 -> Sum4/3
  Product4/1 -> Sum4/2
  Sum4/1 -> "ics "/1

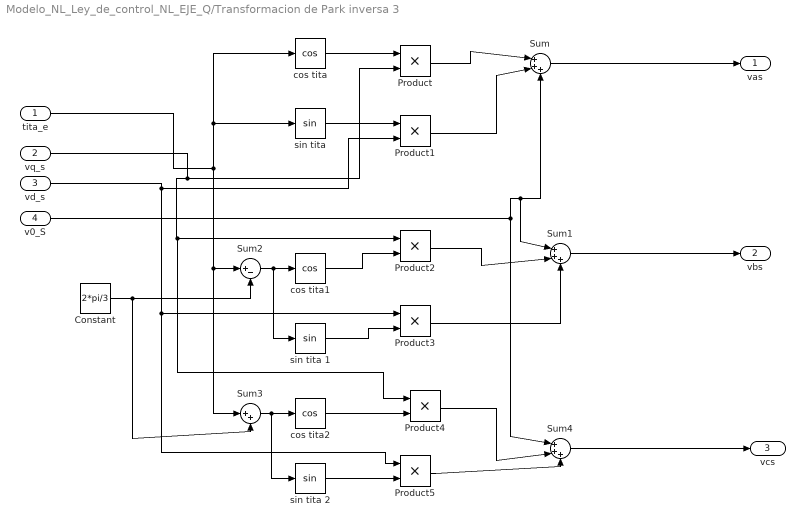
== system Modelo_NL_Ley_de_control_NL_EJE_Q/Transformacion de Park inversa 3 ==
  tita_e : Inport
  vq_s : Inport  Port=2
  vd_s : Inport  Port=3
  "v0_S " : Inport  Port=4
  Constant : Constant  Value=2*pi/3
  Product{,1..5} (6 alike) : Product
  Sum : Sum  Inputs=|+++
  Sum1 : Sum  Inputs=|+++
  Sum2 : Sum  Inputs=|+-
  Sum3 : Sum  Inputs=|++
  Sum4 : Sum  Inputs=|+++
  cos tita : Trigonometry  Operator=cos
  cos tita1 : Trigonometry  Operator=cos
  cos tita2 : Trigonometry  Operator=cos
  "sin tita " : Trigonometry
  sin tita 1 : Trigonometry
  sin tita 2 : Trigonometry
  vas : Outport
  vbs : Outport  Port=2
  "vcs " : Outport  Port=3
  wires:
  tita_e/1 -> Sum3/1, Sum2/1, cos tita/1, "sin tita "/1
  vq_s/1 -> Product4/1, Product2/1, Product/2
  cos tita/1 -> Product/1
  "sin tita "/1 -> Product1/1
  vd_s/1 -> Product5/1, Product3/1, Product1/2
  Product/1 -> Sum/1
  Product1/1 -> Sum/2
  Sum/1 -> vas/1
  "v0_S "/1 -> Sum1/1, Sum/3, Sum4/1
  cos tita1/1 -> Product2/2
  sin tita 1/1 -> Product3/2
  Product3/1 -> Sum1/3
  Product2/1 -> Sum1/2
  Sum1/1 -> vbs/1
  Constant/1 -> Sum3/2, Sum2/2
  Sum2/1 -> sin tita 1/1, cos tita1/1
  Sum3/1 -> sin tita 2/1, cos tita2/1
  cos tita2/1 -> Product4/2
  sin tita 2/1 -> Product5/2
  Product5/1 -> Sum4/3
  Product4/1 -> Sum4/2
  Sum4/1 -> "vcs "/1

== system Modelo_NL_Ley_de_control_NL_EJE_Q/Vq*-1 ==
  Demux : Demux  Tag=STV Demux  Outputs=1
  FromWs : FromWorkspace  Tag=STV FromWs  VariableName=tuvar  SampleTime=0
      SigBuilderData=|
      | common.afterFinalStr = 'Extrapolate'
      | common.sampleTime = 0
      | dataSet.timeRange = [0 2]
      | dataSet.name = 'Group 1'
      | sbobj.Groups.Name = 'Group 1'
      | sbobj.Groups.Signals.Name = 'Signal 1'
      | sbobj.Groups.Signals.XData = [0 0.096 0.096 0.7 0.7 2]
      | sbobj.Groups.Signals.YData = [0 0 19.56 19.56 0 0]
      | sbobj.Groups.TimeRange = [0 2]
  Signal 1 : Outport  Tag=STV Outport
  wires:
  Demux/1 -> Signal 1/1
  FromWs/1 -> Demux/1

== system Modelo_NL_Ley_de_control_NL_EJE_Q/Vq*-2 ==
  Demux : Demux  Tag=STV Demux  Outputs=1
  FromWs : FromWorkspace  Tag=STV FromWs  VariableName=tuvar  SampleTime=0
      SigBuilderData=|
      | common.afterFinalStr = 'Extrapolate'
      | common.sampleTime = 0
      | dataSet.timeRange = [0 2]
      | dataSet.name = 'Group 1'
      | sbobj.Groups.Name = 'Group 1'
      | sbobj.Groups.Signals.Name = 'Signal 1'
      | sbobj.Groups.Signals.XData = [0 0.096 0.096 0.7 0.7 2]
      | sbobj.Groups.Signals.YData = [0 0 19.56 19.56 0 0]
      | sbobj.Groups.TimeRange = [0 2]
  Signal 1 : Outport  Tag=STV Outport
  wires:
  Demux/1 -> Signal 1/1
  FromWs/1 -> Demux/1

== system Modelo_NL_Ley_de_control_NL_EJE_Q/Modelo físico (subsistema electromagnético + mecanico)/Eq 1 ==
  vqrs : Inport
  "Producto 1 " : Inport  Port=2
  Rs : Inport  Port=3
  Gain : Gain  Gain=1/Lq
  Integrator : Integrator
  Product : Product
  Sum : Sum  Inputs=+--
  "iqrs " : Outport
  wires:
  Gain/1 -> Integrator/1
  Sum/1 -> Gain/1
  vqrs/1 -> Sum/1
  Product/1 -> Sum/2
  "Producto 1 "/1 -> Sum/3
  Integrator/1 -> Product/1, "iqrs "/1  "i_qs"
  Rs/1 -> Product/2

== system Modelo_NL_Ley_de_control_NL_EJE_Q/Modelo físico (subsistema electromagnético + mecanico)/Eq 2  ==
  "vdrs " : Inport
  "Producto 2 " : Inport  Port=2
  Rs 1 : Inport  Port=3
  Gain2 : Gain  Gain=1/Ld
  Integrator1 : Integrator
  Product : Product
  Sum1 : Sum  Inputs=|+-+
  "idrs " : Outport
  wires:
  "Producto 2 "/1 -> Sum1/3
  Gain2/1 -> Integrator1/1
  Product/1 -> Sum1/2
  Sum1/1 -> Gain2/1
  Integrator1/1 -> Product/1, "idrs "/1  "i_ds"
  "vdrs "/1 -> Sum1/1
  Rs 1/1 -> Product/2

== system Modelo_NL_Ley_de_control_NL_EJE_Q/Modelo físico (subsistema electromagnético + mecanico)/Eq 3 ==
  "v0rs " : Inport
  Rs 1 : Inport  Port=2
  Gain12 : Gain
  Integrator5 : Integrator
  Producto 1 : Product
  Sum4 : Sum  Inputs=|++
  "i0rs " : Outport
  wires:
  Gain12/1 -> Integrator5/1
  Sum4/1 -> Gain12/1
  Producto 1/1 -> Sum4/2
  "v0rs "/1 -> Sum4/1
  Integrator5/1 -> Producto 1/1, "i0rs "/1  "i_0s"

== system Modelo_NL_Ley_de_control_NL_EJE_Q/Modelo físico (subsistema electromagnético + mecanico)/Signal Builder ==
  Demux : Demux  Tag=STV Demux  Outputs=1
  FromWs : FromWorkspace  Tag=STV FromWs  VariableName=tuvar  SampleTime=0
      SigBuilderData=|
      | common.afterFinalStr = 'Extrapolate'
      | common.sampleTime = 0
      | dataSet.timeRange = [0 2]
      | dataSet.name = 'Group 1'
      | sbobj.Groups.Name = 'Group 1'
      | sbobj.Groups.Signals.Name = 'Signal 2'
      | sbobj.Groups.Signals.XData = [0 0.3 0.3 0.5 0.5 0.9 0.9 2]
      | sbobj.Groups.Signals.YData = [0 0 0.02 0.02 -0.02 -0.02 0 0]
      | sbobj.Groups.TimeRange = [0 2]
  Signal 2 : Outport  Tag=STV Outport
  wires:
  FromWs/1 -> Demux/1
  Demux/1 -> Signal 2/1

== system Modelo_NL_Ley_de_control_NL_EJE_Q/Modelo físico (subsistema electromagnético + mecanico)/Subsistema mecánico ==
  "Tleq " : Inport
  "Tmotor " : Inport  Port=2
  Gain6 : Gain  Gain=1/Jeq
  Gain8 : Gain  Gain=beq
  Integrator3 : Integrator
  Integrator4 : Integrator
  Sum3 : Sum  Inputs=-+-
  "tita_m " : Outport
  "wm " : Outport  Port=2
  Tm : Outport  Port=3
  wires:
  Integrator3/1 -> "tita_m "/1
  Integrator4/1 -> Gain8/1, "wm "/1, Integrator3/1
  Sum3/1 -> Tm/1, Gain6/1
  Gain6/1 -> Integrator4/1
  Gain8/1 -> Sum3/3
  "Tleq "/1 -> Sum3/1
  "Tmotor "/1 -> Sum3/2

== system Modelo_NL_Ley_de_control_NL_EJE_Q/Modelo físico (subsistema electromagnético + mecanico)1/Eq 1 ==
  vqrs : Inport
  "Producto 1 " : Inport  Port=2
  Rs : Inport  Port=3
  Gain : Gain  Gain=1/Lq
  Integrator : Integrator
  Product : Product
  Sum : Sum  Inputs=+--
  "iqrs " : Outport
  wires:
  Gain/1 -> Integrator/1
  Sum/1 -> Gain/1
  vqrs/1 -> Sum/1
  Product/1 -> Sum/2
  "Producto 1 "/1 -> Sum/3
  Integrator/1 -> Product/1, "iqrs "/1  "i_qs"
  Rs/1 -> Product/2

== system Modelo_NL_Ley_de_control_NL_EJE_Q/Modelo físico (subsistema electromagnético + mecanico)1/Eq 2  ==
  "vdrs " : Inport
  "Producto 2 " : Inport  Port=2
  Rs 1 : Inport  Port=3
  Gain2 : Gain  Gain=1/Ld
  Integrator1 : Integrator
  Product : Product
  Sum1 : Sum  Inputs=|+-+
  "idrs " : Outport
  wires:
  "Producto 2 "/1 -> Sum1/3
  Gain2/1 -> Integrator1/1
  Product/1 -> Sum1/2
  Sum1/1 -> Gain2/1
  Integrator1/1 -> Product/1, "idrs "/1  "i_ds"
  "vdrs "/1 -> Sum1/1
  Rs 1/1 -> Product/2

== system Modelo_NL_Ley_de_control_NL_EJE_Q/Modelo físico (subsistema electromagnético + mecanico)1/Eq 3 ==
  "v0rs " : Inport
  Rs 1 : Inport  Port=2
  Gain12 : Gain
  Integrator5 : Integrator
  Producto 1 : Product
  Sum4 : Sum  Inputs=|++
  "i0rs " : Outport
  wires:
  Gain12/1 -> Integrator5/1
  Sum4/1 -> Gain12/1
  Producto 1/1 -> Sum4/2
  "v0rs "/1 -> Sum4/1
  Integrator5/1 -> Producto 1/1, "i0rs "/1  "i_0s"

== system Modelo_NL_Ley_de_control_NL_EJE_Q/Modelo físico (subsistema electromagnético + mecanico)1/Signal Builder ==
  Demux : Demux  Tag=STV Demux  Outputs=1
  FromWs : FromWorkspace  Tag=STV FromWs  VariableName=tuvar  SampleTime=0
      SigBuilderData=|
      | common.afterFinalStr = 'Extrapolate'
      | common.sampleTime = 0
      | dataSet.timeRange = [0 2]
      | dataSet.name = 'Group 1'
      | sbobj.Groups.Name = 'Group 1'
      | sbobj.Groups.Signals.Name = 'Signal 2'
      | sbobj.Groups.Signals.XData = [0 0.3 0.3 0.5 0.5 0.9 0.9 2]
      | sbobj.Groups.Signals.YData = [0 0 0.02 0.02 -0.02 -0.02 0 0]
      | sbobj.Groups.TimeRange = [0 2]
  Signal 2 : Outport  Tag=STV Outport
  wires:
  FromWs/1 -> Demux/1
  Demux/1 -> Signal 2/1

== system Modelo_NL_Ley_de_control_NL_EJE_Q/Modelo físico (subsistema electromagnético + mecanico)1/Subsistema mecánico ==
  "Tleq " : Inport
  "Tmotor " : Inport  Port=2
  Gain6 : Gain  Gain=1/Jeq
  Gain8 : Gain  Gain=beq
  Integrator3 : Integrator
  Integrator4 : Integrator
  Sum3 : Sum  Inputs=-+-
  "tita_m " : Outport
  "wm " : Outport  Port=2
  Tm : Outport  Port=3
  wires:
  Integrator3/1 -> "tita_m "/1
  Integrator4/1 -> Gain8/1, "wm "/1, Integrator3/1
  Sum3/1 -> Tm/1, Gain6/1
  Gain6/1 -> Integrator4/1
  Gain8/1 -> Sum3/3
  "Tleq "/1 -> Sum3/1
  "Tmotor "/1 -> Sum3/2
